simulink model "RRpendulum_digtwin_FSFB_BLDC_accelctrl"  (R2025b)
settings: Solver=FixedStepAuto  StartTime=0.0  StopTime=inf  FixedStep=0.001  RelTol=1e-3  EnableMultiTasking=on
PreLoadFcn:
  | clear;
  | 
  | if isempty(matlab.project.rootProject)
  |     openProject('C:/Users/u0130154/MATLAB/projects/digtwin_labo/digtwin_labo.prj');
  | end
  | prj = matlab.project.rootProject;
  | 
  | %% Define required files
  | dataFolder = fullfile(prj.RootFolder, 'data');
  | 
  | requiredFiles = {
  |     fullfile(dataFolder, 'RRpendulum_params_BLDC.mat')
  |     fullfile(dataFolder, 'FSFB_accel_design.mat')
  |     fullfile(dataFolder, 'UKF_design.mat')
  |     fullfile(dataFolder, 'swingup_design.mat')
  |     fullfile(dataFolder, 'axis1acc_design.mat')
  | };
  | 
  | %% Check if all files exist
  | filesExist = cellfun(@isfile, requiredFiles);
  | 
  | if ~all(filesExist)
  |     fprintf('Some required .mat files are missing. Generating them now...\n');
  | 
  |     % Run generator script (must be on path)
  |     RRpendulum_BLDC_genAllParams;
  | 
  |     % Optional: re-check and error if still missing
  |     dataFolder = fullfile(prj.RootFolder, 'data');
  | requiredFiles = {
  |     fullfile(dataFolder, 'RRpendulum_params_BLDC.mat')
  |     fullfile(dataFolder, 'FSFB_accel_design.mat')
  |     fullfile(dataFolder, 'UKF_design.mat')
  |     fullfile(dataFolder, 'swingup_design.mat')
  |     fullfile(dataFolder, 'axis1acc_design.mat')
  | };
  |     filesExist = cellfun(@isfile, requiredFiles);
  |     if ~all(filesExist)
  |         error('Failed to generate all required .mat files.');
  |     end
  | end
  | 
  | %% Now safely load everything
  | load(requiredFiles{1}, 'params');
  | load(requiredFiles{2}, 'design_accel');
  | fsf_par = design_accel.par;
  | 
  | load(requiredFiles{3}, 'ukf');
  | ukf_par = ukf.par;
  | 
  | load(requiredFiles{4}, 'swingup');
  | swingup_par = swingup.par;
  | load(requiredFiles{5}, 'axis1acc');
  | axis1acc_par = axis1acc.par;
InitFcn:
  | if isempty(matlab.project.rootProject)
  |     openProject('C:/Users/u0130154/MATLAB/projects/digtwin_labo/digtwin_labo.prj');
  | end
  | prj = matlab.project.rootProject;
  | 
  | %% Physical parameters
  | load(fullfile(prj.RootFolder, 'data', 'RRpendulum_params_BLDC.mat'), 'params');
  | 
  | %% Controller design (LQR gains)
  | load(fullfile(prj.RootFolder, 'data', 'FSFB_accel_design.mat'), 'design_accel');
  | fsf_par = design_accel.par;
  | 
  | %% UKF observer design
  | load(fullfile(prj.RootFolder, 'data', 'UKF_design.mat'), 'ukf');
  | ukf_par = ukf.par;
  | 
  | %% Swing-up design (Astrom-Furuta energy controller)
  | load(fullfile(prj.RootFolder, 'data', 'swingup_design.mat'), 'swingup');
  | swingup_par = swingup.par;
  | 
  | %% Acceleration controller
  | load(fullfile(prj.RootFolder, 'data', 'axis1acc_design.mat'), 'axis1acc');
  | axis1acc_par = axis1acc.par;
model workspace (MAT data in the model file):
  COUNTS_PER_TURN_MOT = 8192
  COUNTS_PER_TURN_PEND = 2400
  MOTOR_VEL_RESOLUTION_DIV = 4
  PEND_VEL_RESOLUTION_DIV = 1
  T_SAMPLE = 0.001
undefined symbols (not defined in the file): params
libraries: simulink x4, raspberrypiBasiclib x2, digtwin_labo_lib x1
(part 2 of 2)

== matlab function RRpendulum_digtwin_FSFB_BLDC_accelctrl/Hybrid Controller ==
  settings: updateMethod=DISCRETE
  data: q1_des_in input; x_hat input; alpha1 output; swingup_par parameter; start input; reset input; initstate input; mode_out output; k_e_in input; tau_cv input; fsf_par parameter
function [alpha1, mode_out] = hybrid_swingup_controller(q1_des_in, x_hat, swingup_par, start, reset, initstate, k_e_in, tau_cv, fsf_par)
%#codegen
% Three-phase hybrid controller: swing-up -> stabilize -> FSFB+trajectory
% Output: alpha1 [rad/s^2] — always acceleration, fed to ctrl_axis1_acc

persistent mode q1_ref q1_des dwell_count dropped_count mode_count
if isempty(mode)
    mode = int8(initstate);          % 0=off, 1=stabilize, 2=FSFB+trajectory, 3=swing-up, 4=damping
    q1_ref = 0.0;
    q1_des = 0.0;
    dwell_count = uint32(0);
    dropped_count = uint32(0);
    mode_count = uint32(0);
end

% --- Unpack parameters ---
k_e = k_e_in;
alpha_max = swingup_par.energy.alpha_max;
E0 = swingup_par.energy.E0;
q2_catch = swingup_par.catch.q2_threshold;
E_catch = swingup_par.catch.E_threshold;
m = swingup_par.plant.m;
l = swingup_par.plant.l;
g = swingup_par.plant.g;
r = swingup_par.plant.r;
Kd = fsf_par.lqr.Kd;
Nbar = fsf_par.Nbar;
max_rate = swingup_par.trajectory.max_rate;
Ts = fsf_par.Ts;
E_latch = swingup_par.catch.E_latch;
N_dwell = int32(swingup_par.catch.N_dwell);

q1 = x_hat(1); v1 = x_hat(2); q2 = x_hat(3); v2 = x_hat(4);

% --- Wrap q2 into [0, 2*pi), compute signed error from pi ---
q2_err_signed = wrapTo2Pi(q2)-pi;

% --- Pendulum energy (cos is 2pi-periodic, no wrap needed) ---
%at low acceleration stability depends on which terms are included in E,
%especially v1 components impact convergence
E = 0.5 * m * l^2 * v2^2 - m * g * l * (cos(q2) + 1);
% E = 0.5*(m*r^2 + m*l^2*sin(q2)^2)*v1^2 ...
%     + m*l*r*cos(q2)*v1*v2 ...
%     + 0.5*m*l^2*v2^2 ...
%     - m*g*l*(cos(q2) + 1);
% E = 0.5*m*l*r*cos(q2)*v1*v2 ...
%     + 0.5*m*l^2*v2^2 ...
%     - m*g*l*(cos(q2) + 1);

% --- Catch condition (swing-up -> stabilize) ---
in_catch = (abs(q2_err_signed) < q2_catch) && (abs(E) < E_catch);

if mode == 3 && in_catch
    mode = int8(1);  % enter stabilize phase
end

if reset
    mode = int8(4);  % damping, then turn off
    mode_count = uint32(0);
end

if tau_cv < -0.32 % error reported
    mode = int8(0);  % turn off instantly
    mode_count = uint32(0);
end


if mode == int8(2)
    % === MODE 2: FSFB with q1 trajectory ===
    % Ramp q1_ref
    step = max_rate * Ts;
    err_q1_ref = - q1_ref;
    if err_q1_ref > step
        q1_ref = q1_ref + step;
    elseif err_q1_ref < -step
        q1_ref = q1_ref - step;
    else
        q1_ref = 0;
    end

    % If ref ramped to 0, Ramp q1_des
    if q1_ref == 0
        err_q1 = q1_des_in - q1_des;
        if err_q1 > step
            q1_des = q1_des + step;
        elseif err_q1 < -step
            q1_des = q1_des - step;
        else
            q1_des = q1_des_in;
        end
    else
        q1_des = q1_ref;
    end

    dx = [q1 - q1_ref; v1; q2_err_signed; v2];
    alpha1 = Nbar * (q1_des-q1_ref) - Kd * dx;

    % Count consecutive samples with not(in_catch)
    if ~in_catch
        dropped_count = dropped_count + uint32(1);
    else
        dropped_count = uint32(0);
    end

    if dropped_count > 500
        mode = int8(0);
        mode_count = uint32(0);
    end

elseif mode == int8(1)
    % === MODE 1: Stabilize (no q1 feedback) ===
    dx_partial = [0; v1; q2_err_signed; v2];
    alpha1 = -Kd * dx_partial;
    % Count consecutive samples with |E| < E_latch
    if abs(E) < E_latch
        dwell_count = dwell_count + uint32(1);
    else
        dwell_count = uint32(0);
    end

    % Transition to mode 2 when dwell satisfied
    if dwell_count >= N_dwell
        mode = int8(2);
        mode_count = uint32(0);
        q1_ref = q1;  % latch q1 NOW
    end

    % Count consecutive samples with not(in_catch)
    if ~in_catch
        dropped_count = dropped_count + uint32(1);
    else
        dropped_count = uint32(0);
    end

    if dropped_count > 500
        mode = int8(4);
        mode_count = uint32(0);
    end

elseif mode == int8(3)
    % === MODE 3: Swing-up (energy control, already outputs acceleration) ===
    E_err = E - E0;
    coupling = v2 * cos(q2);
    if coupling > 0, s = 1.0;
    elseif coupling < 0, s = -1.0;
    else, s = 0.0; end
    alpha1 = k_e * E_err * s;
    if alpha1 > alpha_max, alpha1 = alpha_max;
    elseif alpha1 < -alpha_max, alpha1 = -alpha_max; end

elseif mode == int8(4)
    % === MODE 4: damping (gentle velocity brake) ===
    alpha1 = -v1 * 2.0;
    if mode_count >= uint32(8000)
        mode = int8(0);
        mode_count = uint32(0);
    else
        mode_count = mode_count + uint32(1);
    end
else
    % === MODE 0: Off ===
    alpha1 = 0;
    if start %positive flank on run
        mode = int8(3);
    end

end
mode_out = mode;

== matlab function RRpendulum_digtwin_FSFB_BLDC_accelctrl/UKF Observer ==
  settings: updateMethod=DISCRETE  sampleTime=ukf_par.Ts
  data: u input size=1; x_hat output size=[4 1]; y input size=[2 1]; ukf_par parameter
function x_hat = UKF_Observer(u, y, ukf_par)
%#codegen
    persistent x_est P_est isInit

    ukf_Q       = ukf_par.noise.Q;
    ukf_R       = ukf_par.noise.R;
    ukf_Wm      = ukf_par.sigma.Wm;
    ukf_Wc      = ukf_par.sigma.Wc;
    ukf_lambda  = ukf_par.sigma.lambda;
    ukf_C       = ukf_par.measurement.C;
    ukf_Ts      = ukf_par.Ts;
    ukf_x0      = ukf_par.ic.x0;
    ukf_P0      = ukf_par.ic.P0;


    if isempty(isInit)
        x_est = zeros(4,1);
        P_est = zeros(4,4);
        x_est(:) = ukf_x0;
        P_est(:) = ukf_P0;
        isInit = true;
    end

    x_new = zeros(4,1);
    P_new = zeros(4,4);
    [x_new, P_new] = ukf_observer_step(x_est, P_est, u, y, ...
        ukf_Q, ukf_R, ukf_Wm, ukf_Wc, ukf_lambda, ukf_C, ukf_Ts);
    x_est = x_new;
    P_est = P_new;

    x_hat = x_est;
end

== matlab function RRpendulum_digtwin_FSFB_BLDC_accelctrl/acceleration controller ==
  data: x_hat input; tau_a output; qa_dd_ref input; vref_state input; vref_out output; params parameter; axis1acc_par parameter
function [tau_a, vref_out] = ctrl_axis1_acc( ...
        x_hat, qa_dd_ref, vref_state, params, axis1acc_par)
%#codegen

    p = params.mech;
    ctrl = axis1acc_par;
    q = x_hat([1,3]);
    v = x_hat([2,4]);

    Meff = compute_Meff(q, p.Iz_1, p.l, p.m, p.r);
    h    = compute_h(q, v, p.Iz_1, p.l, p.m, p.r, p.b1, p.b2, p.g);

    % Integral of acceleration error, rewritten using UKF velocity:
    %   int = ∫(qa_dd_ref - qa_dd_hat) dt  ==  vref - v_hat_a
    err_int = vref_state - v(1);

    % Inverse-dynamics feedforward + I action
    tau_unsat = Meff*(qa_dd_ref + ctrl.Ki*err_int) + h;
    tau_a     = min(max(tau_unsat, ctrl.tau_min), ctrl.tau_max);

    % Update virtual reference velocity (integrate ref accel + AW back-calc)
    Kaw      = 1/ctrl.tau_f_aw;
    vref_out = vref_state + ctrl.Ts*(qa_dd_ref + Kaw*(tau_a - tau_unsat)/Meff);
end

== stateflow chart RRpendulum_digtwin_FSFB_BLDC_accelctrl/Chart ==
  state wait
    sp_out = 0;
  state Stabilize
    state stabilized0
      sp_out = sp_in;
    state stabilized1
      sp_out = sp_in + 0.25;
    state stabilized3
      sp_out = sp_in - 0.25;
    state stabilized2
      sp_out = sp_in;
    (default) -> stabilized0
    stabilized0 -> stabilized1 : after(0.5,'sec') [start]
    stabilized3 -> stabilized0 : after(0.5,'sec') [start]
    stabilized1 -> stabilized2 : after(0.5,'sec') [start]
    stabilized2 -> stabilized3 : after(0.5,'sec') [start]
  (default) -> wait
  Stabilize -> wait : [mode ~= 2]
  wait -> Stabilize : [mode == 2]
  data: sp_in input; sp_out output; start input; mode input
